simulink model "tank_drive"  (R2021a)
settings: Solver=ode3  StartTime=0.0  StopTime=inf  RelTol=1e-3  EnableMultiTasking=on
libraries: vexv5lib x18, vexcommonlib x1
settings Model: ExtModeTrigDuration=25  Creator=dbayl  LastModifiedBy=dbayl
settings SolverCC: AlgebraicLoopSolver=TrustRegion
settings DataIOCC: LimitDataPoints=on  SaveFormat=Array
settings OptimizationCC: ExpressionDepthLimit=2147483647  LifeSpan=Inf  MaxStackSize=64
settings DebuggingCC: UnderspecifiedInitializationDetection=Classic  MergeDetectMultiDrivingBlocksExec=none  InheritedTsInSrcMsg=none  FcnCallInpInsideContextMsg=warning  UnconnectedInputMsg=none  UnconnectedOutputMsg=none  AllowSymbolicDim=off  StateNameClashWarn=warning  PregeneratedLibrarySubsystemCodeDiagnostic=none  SFUnexpectedBacktrackingDiag=warning  SFNoUnconditionalDefaultTransitionDiag=warning  SFExecutionAtInitializationDiag=none  SFMachineParentedDataDiag=warning  ArithmeticOperatorsInVariantConditions=warning
settings HardwareCC: ProdBitPerPointer=32  ProdBitPerSizeT=32  ProdBitPerPtrDiffT=32  ProdLargestAtomicInteger=Long  ProdLargestAtomicFloat=Double  ProdWordSize=32  ProdHWDeviceType=ARM Compatible->ARM Cortex  UseEmbeddedCoderFeatures=off
settings ModelReferenceCC: PropagateSignalLabelsOutOfModel=off
settings SFSimCC: SimUseLocalCustomCode=off  CustomCodeUndefinedFunction=UseInterfaceOnly
settings RTWCC: SystemTargetFile=ert.tlc  HardwareBoard=VEX V5 Robot Brain  TLCOptions=-aInlineSetEventsForThisBaseRateFcn=TLC_FALSE -aSuppressMultiTaskScheduler=TLC_FALSE -aRateBasedStepFcn=0  TemplateMakefile=ert_default_tmf  RTWUseLocalCustomCode=off  Toolchain=GNU Tools for ARM Embedded Processors
settings CodeAppCC: StateflowObjectComments=on
settings ERTTargetCC: CodeReplacementLibrary=GCC ARM Cortex-M3  MultiwordLength=2048  ERTCustomFileBanners=off  SupportContinuousTime=on  SupportNonInlinedSFcns=on  RemoveResetFunc=off  ModelStepFunctionPrototypeControlCompliant=off  ConvertIfToSwitch=off  SuppressUnreachableDefaultCases=off
settings ConfigComp: CovMetricSettings=dw  CovSaveCumulativeToWorkspaceVar=on  CovSaveSingleToWorkspaceVar=on  CovExternalEMLEnable=off  CovSFcnEnable=off

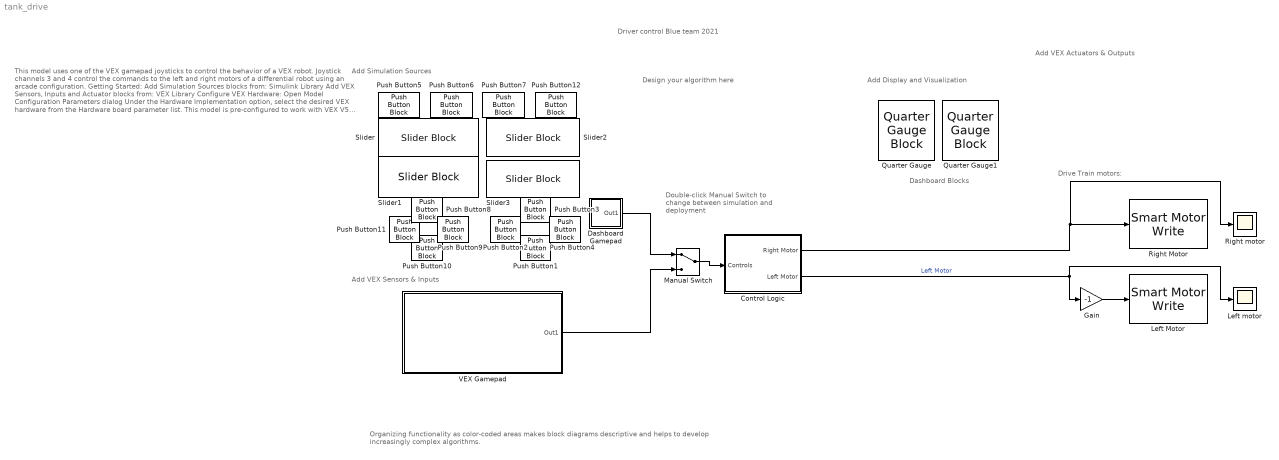
== system tank_drive ==
  note: Add VEX Actuators & Outputs
  note: Dashboard Blocks
  note: Driver control Blue team 2021
  note: This model uses one of the VEX gamepad joysticks to control the behavior of a VEX robot.
      | Joystick channels 3 and 4 control the commands to the left and right motors of a differential robot using an arcade configuration.
      |
      | Getting Started:
      |
      | Add Simulation Sources blocks from:
      | Simulink Library
      | Add VEX Sensors, Inputs and Actuator blocks from:
      | VEX Library
      |
      | Configure VEX Hardware:
      |
      | Open Model Configuration Parameters dialog
      | Under the Hardware Implementation option, select the desired VEX hardware from the Hardware board parameter list.
      |
      | This model is pre-configured to work with VEX V5 Robot Brain.
      |
      | Simulate the Model
      |
      | Click the Run button on the Simulation Tab in Simulink Toolstrip.
      |
      | Run the Model on VEX Hardware
      |
      | Click the Build, Deploy & Start button on Hardware Tab in Simulink Toolstrip.
  note: Add VEX Sensors & Inputs
  note: Design your algorithm here
  note: Add Display and Visualization
  note: Organizing functionality as color-coded areas makes block diagrams descriptive and helps to develop increasingly complex algorithms.
  note: Add Simulation Sources
  note: Drive Train motors:
  note: Double-click Manual Switch
      | to change between simulation
      | and deployment
  Control Logic : Subsystem
  Dashboard Gamepad : Subsystem
  Gain : Gain  Gain=-1
  Left Motor : vexv5lib/Actuators/Smart Motor Write  motorPort=2  scaleFactor=36:1  MotorBrakeMode=Coast  OperationMode=Velocity Control
      settings: SourceProductBaseCode=VEXV5
  Left motor : Scope
  Manual Switch : ManualSwitch
  Push Button1 : PushButtonBlock  ButtonText=B
  Push Button10 : PushButtonBlock  ButtonText=v
  Push Button11 : PushButtonBlock  ButtonText=<
  Push Button12 : PushButtonBlock  ButtonText=R2
  Push Button2 : PushButtonBlock  ButtonText=Y
  Push Button3 : PushButtonBlock  ButtonText=X
  Push Button4 : PushButtonBlock  ButtonText=A
  Push Button5 : PushButtonBlock  ButtonText=L1
  Push Button6 : PushButtonBlock  ButtonText=L2
  Push Button7 : PushButtonBlock  ButtonText=R1
  Push Button8 : PushButtonBlock  ButtonText=^
  Push Button9 : PushButtonBlock  ButtonText=>
  Quarter Gauge : QuarterGaugeBlock  ScaleMin=-128  ScaleMax=127
  Quarter Gauge1 : QuarterGaugeBlock  ScaleMin=-128  ScaleMax=127
  Right Motor : vexv5lib/Actuators/Smart Motor Write  motorPort=1  scaleFactor=36:1  MotorBrakeMode=Coast  OperationMode=Velocity Control
      settings: SourceProductBaseCode=VEXV5
  Right motor : Scope
  Slider{,1..3} (4 alike) : SliderBlock  ScaleMin=-128  ScaleMax=127
  VEX Gamepad : Subsystem
  wires:
  Manual Switch/1 -> Control Logic/1(Controls)
  Dashboard Gamepad/1(Out1) -> Manual Switch/1
  VEX Gamepad/1(Out1) -> Manual Switch/2
  Control Logic/2(Left Motor) -> Gain/1, Left motor/1  "Left Motor"
  Gain/1 -> Left Motor/1
  Control Logic/1(Right Motor) -> Right motor/1, Right Motor/1

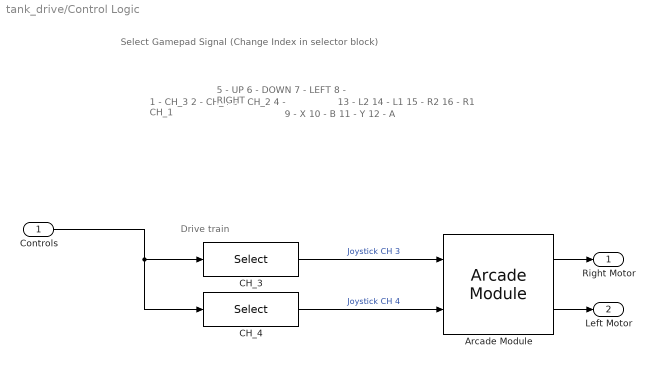
== system tank_drive/Control Logic ==
  note: Drive train
  note: 1 - CH_3
      | 2 - CH_4
      | 3 - CH_2
      | 4 - CH_1
  note: Select Gamepad Signal
      | (Change Index in selector block)
  note: 5 - UP
      | 6 - DOWN
      | 7 - LEFT
      | 8 - RIGHT
  note: 9   - X
      | 10 - B
      | 11 - Y
      | 12 - A
  note: 13 - L2
      | 14 - L1
      | 15 - R2
      | 16 - R1
  Controls : Inport
  Arcade Module : vexcommonlib/Arcade Module  BlockPlatform=vexarmcortex
      settings: SourceProductBaseCode=EC_VEX_MICRO,VEXV5
  CH_3 : Selector  InputPortWidth=16  IndexOptions=Index vector (dialog)  Indices=1  OutputSizes=1
  CH_4 : Selector  InputPortWidth=16  IndexOptions=Index vector (dialog)  Indices=2  OutputSizes=1
  Right Motor : Outport  VectorParamsAs1DForOutWhenUnconnected=off
  Left Motor : Outport  Port=2  VectorParamsAs1DForOutWhenUnconnected=off
  wires:
  Controls/1 -> CH_4/1, CH_3/1
  CH_3/1 -> Arcade Module/1  "Joystick CH 3"
  CH_4/1 -> Arcade Module/2  "Joystick CH 4"
  Arcade Module/1 -> Right Motor/1
  Arcade Module/2 -> Left Motor/1

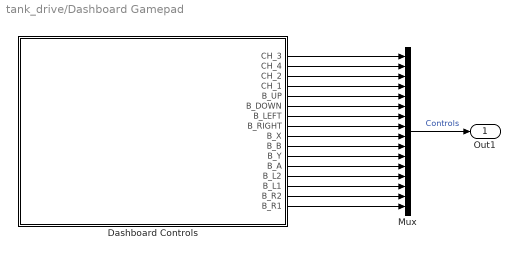
== system tank_drive/Dashboard Gamepad ==
  Dashboard Controls : Subsystem
  Mux : Mux  Inputs=16
  Out1 : Outport  VectorParamsAs1DForOutWhenUnconnected=off
  wires:
  Dashboard Controls/12(B_A) -> Mux/12
  Dashboard Controls/16(B_R1) -> Mux/16
  Dashboard Controls/4(CH_1) -> Mux/4
  Dashboard Controls/15(B_R2) -> Mux/15
  Dashboard Controls/6(B_DOWN) -> Mux/6
  Dashboard Controls/11(B_Y) -> Mux/11
  Dashboard Controls/13(B_L2) -> Mux/13
  Dashboard Controls/14(B_L1) -> Mux/14
  Dashboard Controls/3(CH_2) -> Mux/3
  Dashboard Controls/7(B_LEFT) -> Mux/7
  Dashboard Controls/5(B_UP) -> Mux/5
  Dashboard Controls/9(B_X) -> Mux/9
  Dashboard Controls/10(B_B) -> Mux/10
  Dashboard Controls/8(B_RIGHT) -> Mux/8
  Dashboard Controls/1(CH_3) -> Mux/1
  Dashboard Controls/2(CH_4) -> Mux/2
  Mux/1 -> Out1/1  "Controls"

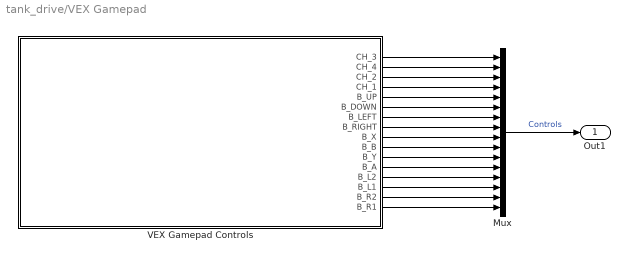
== system tank_drive/VEX Gamepad ==
  Mux : Mux  Inputs=16
  VEX Gamepad Controls : Subsystem
  Out1 : Outport  VectorParamsAs1DForOutWhenUnconnected=off
  wires:
  Mux/1 -> Out1/1  "Controls"
  VEX Gamepad Controls/2(CH_4) -> Mux/2
  VEX Gamepad Controls/1(CH_3) -> Mux/1
  VEX Gamepad Controls/8(B_RIGHT) -> Mux/8
  VEX Gamepad Controls/10(B_B) -> Mux/10
  VEX Gamepad Controls/9(B_X) -> Mux/9
  VEX Gamepad Controls/5(B_UP) -> Mux/5
  VEX Gamepad Controls/7(B_LEFT) -> Mux/7
  VEX Gamepad Controls/3(CH_2) -> Mux/3
  VEX Gamepad Controls/14(B_L1) -> Mux/14
  VEX Gamepad Controls/13(B_L2) -> Mux/13
  VEX Gamepad Controls/11(B_Y) -> Mux/11
  VEX Gamepad Controls/6(B_DOWN) -> Mux/6
  VEX Gamepad Controls/15(B_R2) -> Mux/15
  VEX Gamepad Controls/4(CH_1) -> Mux/4
  VEX Gamepad Controls/16(B_R1) -> Mux/16
  VEX Gamepad Controls/12(B_A) -> Mux/12

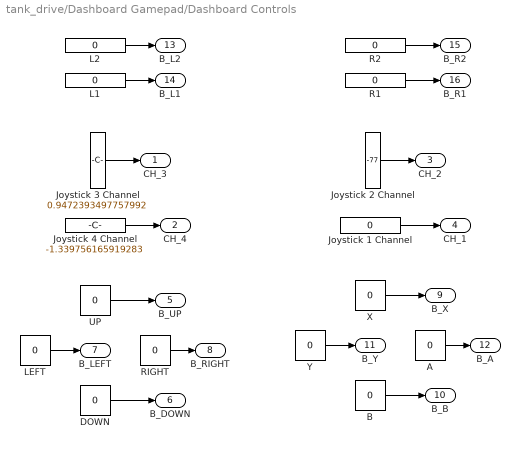
== system tank_drive/Dashboard Gamepad/Dashboard Controls ==
  A : Constant  Value=0
  B : Constant  Value=0
  DOWN : Constant  Value=0
  Joystick 1 Channel : Constant  Value=0
  Joystick 2 Channel : Constant  Value=-77
  Joystick 3 Channel : Constant  Value=0.9472393497757992
  Joystick 4 Channel : Constant  Value=-1.339756165919283
  L1 : Constant  Value=0
  L2 : Constant  Value=0
  LEFT : Constant  Value=0
  R1 : Constant  Value=0
  R2 : Constant  Value=0
  RIGHT : Constant  Value=0
  UP : Constant  Value=0
  X : Constant  Value=0
  Y : Constant  Value=0
  CH_3 : Outport  VectorParamsAs1DForOutWhenUnconnected=off
  CH_4 : Outport  Port=2  VectorParamsAs1DForOutWhenUnconnected=off
  CH_2 : Outport  Port=3  VectorParamsAs1DForOutWhenUnconnected=off
  CH_1 : Outport  Port=4  VectorParamsAs1DForOutWhenUnconnected=off
  B_UP : Outport  Port=5  VectorParamsAs1DForOutWhenUnconnected=off
  B_DOWN : Outport  Port=6  VectorParamsAs1DForOutWhenUnconnected=off
  B_LEFT : Outport  Port=7  VectorParamsAs1DForOutWhenUnconnected=off
  B_RIGHT : Outport  Port=8  VectorParamsAs1DForOutWhenUnconnected=off
  B_X : Outport  Port=9  VectorParamsAs1DForOutWhenUnconnected=off
  B_B : Outport  Port=10  VectorParamsAs1DForOutWhenUnconnected=off
  B_Y : Outport  Port=11  VectorParamsAs1DForOutWhenUnconnected=off
  B_A : Outport  Port=12  VectorParamsAs1DForOutWhenUnconnected=off
  B_L2 : Outport  Port=13  VectorParamsAs1DForOutWhenUnconnected=off
  B_L1 : Outport  Port=14  VectorParamsAs1DForOutWhenUnconnected=off
  B_R2 : Outport  Port=15  VectorParamsAs1DForOutWhenUnconnected=off
  B_R1 : Outport  Port=16  VectorParamsAs1DForOutWhenUnconnected=off
  wires:
  Joystick 3 Channel/1 -> CH_3/1
  Joystick 4 Channel/1 -> CH_4/1
  Joystick 2 Channel/1 -> CH_2/1
  Joystick 1 Channel/1 -> CH_1/1
  UP/1 -> B_UP/1
  DOWN/1 -> B_DOWN/1
  LEFT/1 -> B_LEFT/1
  RIGHT/1 -> B_RIGHT/1
  X/1 -> B_X/1
  B/1 -> B_B/1
  Y/1 -> B_Y/1
  A/1 -> B_A/1
  L2/1 -> B_L2/1
  L1/1 -> B_L1/1
  R2/1 -> B_R2/1
  R1/1 -> B_R1/1

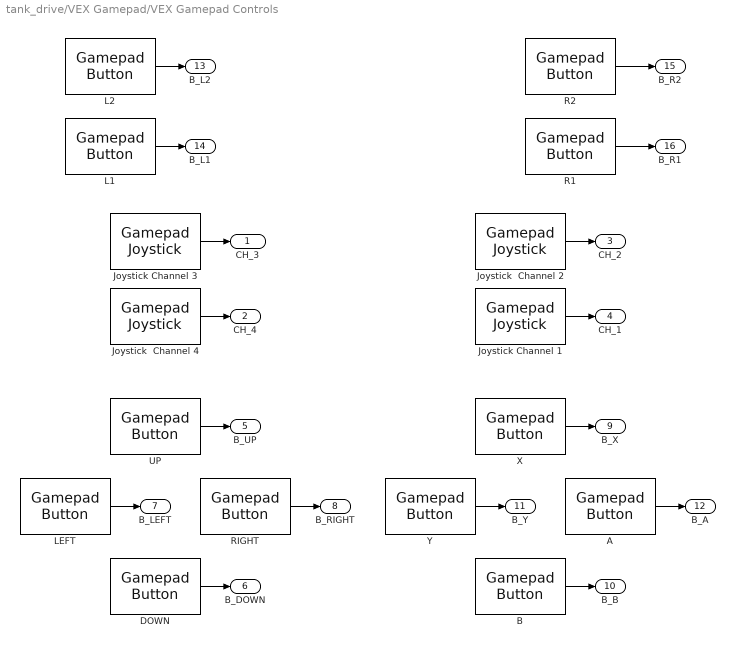
== system tank_drive/VEX Gamepad/VEX Gamepad Controls ==
  A : vexv5lib/Gamepad/Gamepad Button  joystickType=Master  chan=A  SampleTime=0.02
      settings: SourceProductBaseCode=VEXV5
  B : vexv5lib/Gamepad/Gamepad Button  joystickType=Master  chan=B  SampleTime=0.02
      settings: SourceProductBaseCode=VEXV5
  DOWN : vexv5lib/Gamepad/Gamepad Button  joystickType=Master  chan=DOWN  SampleTime=0.02
      settings: SourceProductBaseCode=VEXV5
  Joystick  Channel 2 : vexv5lib/Gamepad/Gamepad Joystick  joystickType=Master  chan=2  SampleTime=0.02
      settings: SourceProductBaseCode=VEXV5
  Joystick  Channel 4 : vexv5lib/Gamepad/Gamepad Joystick  joystickType=Master  chan=4  SampleTime=0.02
      settings: SourceProductBaseCode=VEXV5
  Joystick Channel 1 : vexv5lib/Gamepad/Gamepad Joystick  joystickType=Master  chan=1  SampleTime=0.02
      settings: SourceProductBaseCode=VEXV5
  Joystick Channel 3 : vexv5lib/Gamepad/Gamepad Joystick  joystickType=Master  chan=3  SampleTime=0.02
      settings: SourceProductBaseCode=VEXV5
  L1 : vexv5lib/Gamepad/Gamepad Button  joystickType=Master  chan=L1  SampleTime=0.02
      settings: SourceProductBaseCode=VEXV5
  L2 : vexv5lib/Gamepad/Gamepad Button  joystickType=Master  chan=L2  SampleTime=0.02
      settings: SourceProductBaseCode=VEXV5
  LEFT : vexv5lib/Gamepad/Gamepad Button  joystickType=Master  chan=LEFT  SampleTime=0.02
      settings: SourceProductBaseCode=VEXV5
  R1 : vexv5lib/Gamepad/Gamepad Button  joystickType=Master  chan=R1  SampleTime=0.02
      settings: SourceProductBaseCode=VEXV5
  R2 : vexv5lib/Gamepad/Gamepad Button  joystickType=Master  chan=R2  SampleTime=0.02
      settings: SourceProductBaseCode=VEXV5
  RIGHT : vexv5lib/Gamepad/Gamepad Button  joystickType=Master  chan=RIGHT  SampleTime=0.02
      settings: SourceProductBaseCode=VEXV5
  UP : vexv5lib/Gamepad/Gamepad Button  joystickType=Master  chan=UP  SampleTime=0.02
      settings: SourceProductBaseCode=VEXV5
  X : vexv5lib/Gamepad/Gamepad Button  joystickType=Master  chan=X  SampleTime=0.02
      settings: SourceProductBaseCode=VEXV5
  Y : vexv5lib/Gamepad/Gamepad Button  joystickType=Master  chan=Y  SampleTime=0.02
      settings: SourceProductBaseCode=VEXV5
  CH_3 : Outport  VectorParamsAs1DForOutWhenUnconnected=off
  CH_4 : Outport  Port=2  VectorParamsAs1DForOutWhenUnconnected=off
  CH_2 : Outport  Port=3  VectorParamsAs1DForOutWhenUnconnected=off
  CH_1 : Outport  Port=4  VectorParamsAs1DForOutWhenUnconnected=off
  B_UP : Outport  Port=5  VectorParamsAs1DForOutWhenUnconnected=off
  B_DOWN : Outport  Port=6  VectorParamsAs1DForOutWhenUnconnected=off
  B_LEFT : Outport  Port=7  VectorParamsAs1DForOutWhenUnconnected=off
  B_RIGHT : Outport  Port=8  VectorParamsAs1DForOutWhenUnconnected=off
  B_X : Outport  Port=9  VectorParamsAs1DForOutWhenUnconnected=off
  B_B : Outport  Port=10  VectorParamsAs1DForOutWhenUnconnected=off
  B_Y : Outport  Port=11  VectorParamsAs1DForOutWhenUnconnected=off
  B_A : Outport  Port=12  VectorParamsAs1DForOutWhenUnconnected=off
  B_L2 : Outport  Port=13  VectorParamsAs1DForOutWhenUnconnected=off
  B_L1 : Outport  Port=14  VectorParamsAs1DForOutWhenUnconnected=off
  B_R2 : Outport  Port=15  VectorParamsAs1DForOutWhenUnconnected=off
  B_R1 : Outport  Port=16  VectorParamsAs1DForOutWhenUnconnected=off
  wires:
  L1/1 -> B_L1/1
  X/1 -> B_X/1
  RIGHT/1 -> B_RIGHT/1
  LEFT/1 -> B_LEFT/1
  DOWN/1 -> B_DOWN/1
  UP/1 -> B_UP/1
  Joystick Channel 1/1 -> CH_1/1
  Joystick  Channel 2/1 -> CH_2/1
  Joystick  Channel 4/1 -> CH_4/1
  Joystick Channel 3/1 -> CH_3/1
  L2/1 -> B_L2/1
  R1/1 -> B_R1/1
  R2/1 -> B_R2/1
  B/1 -> B_B/1
  Y/1 -> B_Y/1
  A/1 -> B_A/1
